simulink library "Nokia_Arduino_Blocks"  (Simulink 7.5)
settings: Solver=ode45  StartTime=0.0  StopTime=10.0  RelTol=1e-3
settings Model: Creator=tyler  LastModifiedBy=Wildcat

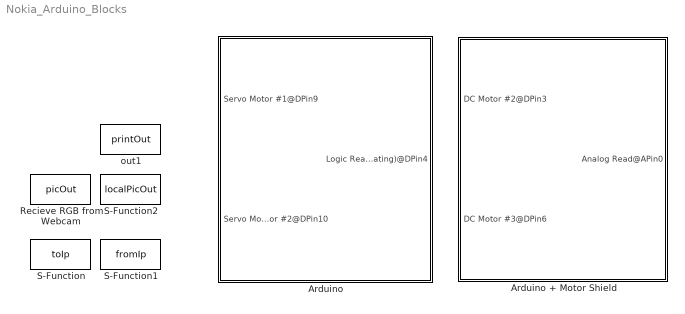
== system Nokia_Arduino_Blocks ==
  Arduino : Subsystem  mask{PinConfig0=Rx, PinConfig1=Tx, PinConfig2=Unused, PinConfig3=Unused, PinConfig4=Logic Read (floating), PinConfig5=Unused, PinConfig6=Unused, PinConfig7=Unused, PinConfig8=Unused, PinConfig9=Servo Motor #1, PinConfig10=Servo Motor #2, PinConfig11=Unused, PinConfig12=Unused, PinConfig13=Unused, ApinConfig0=Unused, ApinConfig1=Unused, ApinConfig2=Unused, ApinConfig3=Unused, ApinConfig4=Unused, ApinConfig5=Unused}
      mask prompts: PinConfig0 "Digital Pin 0 :"; PinConfig1 "Digital Pin 1 :"; PinConfig2 "Digital Pin 2 :"; PinConfig3 "Digital Pin 3 :"; PinConfig4 "Digital Pin 4 :"; PinConfig5 "Digital Pin 5 :"; PinConfig6 "Digital Pin 6 :"; PinConfig7 "Digital Pin 7 :"; PinConfig8 "Digital Pin 8 :"; PinConfig9 "Digital Pin 9 :"; PinConfig10 "Digital Pin 10:"; PinConfig11 "Digital Pin 11:"; PinConfig12 "Digital Pin 12:"; PinConfig13 "Digital Pin 13:"; ApinConfig0 "Analog Input 0:"; ApinConfig1 "Analog Input 1:"; ApinConfig2 "Analog Input 2:"; ApinConfig3 "Analog Input 3:"; ApinConfig4 "Analog Input 4:"; ApinConfig5 "Analog Input 5:"
      mask init:
      | set_param(gcb, 'LinkStatus', 'none')
      | ardInterface('all');
      mask StyleString: popup(Unused|Rx|Logic Write|Logic Read (floating)|Logic Read (pulled high)),popup(Unused|Tx|Logic Write|Logic Read (floating)|Logic Read (pulled high)),popup(Unused|Encoder (with pin 4)|Logic Write|Logic Read (floating)|Logic Read (pulled high)),popup(Unused|Encoder (with pin 5)|PWM Write|Logic Write|Logic Read (floating)|Logic Read (pulled high)),popup(Unused|Logic Write|Logic Read (floating)|Logic Read (pulled high)),popup(Unused|PWM Write|Logic Write|Logic Read (floating)|Logic Read (pulled high)),popup(Unused|PWM Write|Logic Write|Logic Read (floating)|Logic Read (pulled high)),popup(Unused|Logic Write|Logic Read (floating)|Logic Read (pulled high)),popup(Unused|Logic Write|Logic Read (floating)|Logic Read (pulled high)),popup(Unused|PWM Write|Logic Write|Servo Motor #1|Logic Read (floating)|Logic Read (pulled high)),popup(Unused|PWM Write|Logic Write|Servo Motor #2|Logic Read (floating)|Logic Read (pulled high)),popup(Unused|PWM Write|Logic Write|Logic Read (floating)|Logic Read (pulled high)),popup(Unused|PWM Write|Logic Write|Logic Read (floating)|Logic Read (pulled high)),popup(Unused|Logic Write|Logic Read (floating)|Logic Read (pulled high)),popup(Unused|Analog Read),popup(Unused|Analog Read),popup(Unused|Analog Read),popup(Unused|Analog Read),popup(Unused|Analog Read),popup(Unused|Analog Read)
      mask CallbackString:
      | ||ardInterface('clearAll');
      | set_param(gcb, 'LinkStatus', 'none')
      | maskStr = get_param(gcb,'MaskEnables');
      | maskVals = get_param(gcb,'MaskValues');
      | if strcmp(get_param(gcb,'PinConfig2'),'Encoder (with pin 4)')
      |     maskStr{5}='off';
      |     maskVals{5}='Unused';
      | else
      |     maskStr{5}='on';
      | end
      | 
      | set_param(gcb,'MaskEnables',maskStr);
      | set_param(gcb,'MaskValues',maskVals);
      | |ardInterface('clearAll');
      | set_param(gcb, 'LinkStatus', 'none')
      | maskStr = get_param(gcb,'MaskEnables');
      | maskVals = get_param(gcb,'MaskValues');
      | if strcmp(get_param(gcb,'PinConfig3'),'Encoder (with pin 5)')
      |     maskStr{6}='off';
      |     maskVals{6}='Unused';
      | else
      |     maskStr{6}='on';
      | end
      | 
      | set_param(gcb,'MaskEnables',maskStr);
      | set_param(gcb,'MaskValues',maskVals);
      | ||||||||||||||||
      mask TabNameString: Digital I/O,Digital I/O,Digital I/O,Digital I/O,Digital I/O,Digital I/O,Digital I/O,Digital I/O,Digital I/O,Digital I/O,Digital I/O,Digital I/O,Digital I/O,Digital I/O,Analog Output,Analog Output,Analog Output,Analog Output,Analog Output,Analog Output
  Arduino + Motor Shield : Subsystem  mask{PinConfig0=Rx, PinConfig1=Tx, PinConfig2=Unused, PinConfig3=DC Motor #2, PinConfig4=Unused, PinConfig5=Unused, PinConfig6=DC Motor #3, PinConfig7=Unused, PinConfig8=Unused, PinConfig9=Unused, PinConfig10=Unused, PinConfig11=Unused, PinConfig12=Unused, PinConfig13=Unused, ApinConfig0=Analog Read, ApinConfig1=Unused, ApinConfig2=Unused, ApinConfig3=Unused, ApinConfig4=Unused, ApinConfig5=Unused}
      mask prompts: PinConfig0 "Digital Pin 0 :"; PinConfig1 "Digital Pin 1 :"; PinConfig2 "Digital Pin 2 :"; PinConfig3 "Digital Pin 3 :"; PinConfig4 "Digital Pin 4 :"; PinConfig5 "Digital Pin 5 :"; PinConfig6 "Digital Pin 6 :"; PinConfig7 "Digital Pin 7 :"; PinConfig8 "Digital Pin 8 :"; PinConfig9 "Digital Pin 9 :"; PinConfig10 "Digital Pin 10:"; PinConfig11 "Digital Pin 11:"; PinConfig12 "Digital Pin 12:"; PinConfig13 "Digital Pin 13:"; ApinConfig0 "Analog Input 0:"; ApinConfig1 "Analog Input 1:"; ApinConfig2 "Analog Input 2:"; ApinConfig3 "Analog Input 3:"; ApinConfig4 "Analog Input 4:"; ApinConfig5 "Analog Input 5:"
      mask init:
      | set_param(gcb, 'LinkStatus', 'none')
      | ardInterface('all');
      mask StyleString: popup(Unused|Rx|Logic Write|Logic Read (floating)|Logic Read (pulled high)),popup(Unused|Tx|Logic Write|Logic Read (floating)|Logic Read (pulled high)),popup(Unused|Encoder (with pin 9)|Logic Write|Logic Read (floating)|Logic Read (pulled high)),popup(Unused|Encoder (with pin 10)|PWM Write|Logic Write|Logic Read (floating)|Logic Read (pulled high)|DC Motor #2|Stepper Motor #1),popup(Unused|Logic Write|Logic Read (floating)|Logic Read (pulled high)),popup(Unused|PWM Write|Logic Write|Logic Read (floating)|Logic Read (pulled high)|DC Motor #4|Stepper Motor #2),popup(Unused|PWM Write|Logic Write|Logic Read (floating)|Logic Read (pulled high)|DC Motor #3|Stepper Motor #2),popup(Unused|Logic Write|Logic Read (floating)|Logic Read (pulled high)),popup(Unused|Logic Write|Logic Read (floating)|Logic Read (pulled high)),popup(Unused|PWM Write|Logic Write|Logic Read (floating)|Logic Read (pulled high)),popup(Unused|PWM Write|Logic Write|Logic Read (floating)|Logic Read (pulled high)),popup(Unused|PWM Write|Logic Write|Logic Read (floating)|Logic Read (pulled high)|DC Motor #1|Stepper Motor #1),popup(Unused|PWM Write|Logic Write|Logic Read (floating)|Logic Read (pulled high)),popup(Unused|Logic Write|Logic Read (floating)|Logic Read (pulled high)),popup(Unused|Analog Read),popup(Unused|Analog Read),popup(Unused|Analog Read),popup(Unused|Analog Read),popup(Unused|Analog Read),popup(Unused|Analog Read)
      mask CallbackString:
      | ardInterface('clearAll');|ardInterface('clearAll');|ardInterface('clearAll');
      | set_param(gcb, 'LinkStatus', 'none')
      | maskStr = get_param(gcb,'MaskEnables');
      | maskVals = get_param(gcb,'MaskValues');
      | if strcmp(get_param(gcb,'PinConfig2'),'Encoder (with pin 9)')
      |     maskStr{10}='off';
      |     maskVals{10}='Unused';
      | else
      |     maskStr{10}='on';
      | end
      | 
      | set_param(gcb,'MaskEnables',maskStr);
      | set_param(gcb,'MaskValues',maskVals);
      | |ardInterface('clearAll');
      | set_param(gcb, 'LinkStatus', 'none')
      | maskStr = get_param(gcb,'MaskEnables');
      | maskVals = get_param(gcb,'MaskValues');
      | if strcmp(get_param(gcb,'PinConfig3'),'Encoder (with pin 10)')
      |     maskStr{11}='off';
      |     maskVals{11}='Unused';
      | else
      |     maskStr{11}='on';
      | end
      | 
      | if strcmp(get_param(gcb,'PinConfig3'),'Stepper Motor #1')
      |     maskStr{12}='off';
      |     maskVals{12}='Unused';
      | else
      |     maskStr{12}='on';
      | end
      | if (sum(cell2mat(strfind(get_param(gcb,'MaskValues'),'Motor'))))
      | maskStr{5}='off';
      | maskVals{5}='Unused';
      | maskStr{8}='off';
      | maskVals{8}='Unused';
      | maskStr{9}='off';
      | maskVals{9}='Unused';
      | maskStr{13}='off';
      | maskVals{13}='Unused';
      | else
      | maskStr{5}='on';
      | maskStr{8}='on';
      | maskStr{9}='on';
      | maskStr{13}='on';
      | end
      | set_param(gcb,'MaskEnables',maskStr);
      | set_param(gcb,'MaskValues',maskVals);|ardInterface('clearAll');
      | |ardInterface('clearAll');
      | set_param(gcb, 'LinkStatus', 'none')
      | maskStr = get_param(gcb,'MaskEnables');
      | maskVals = get_param(gcb,'MaskValues');
      | if strcmp(get_param(gcb,'PinConfig5'),'Stepper Motor #2')
      |     maskStr{7}='off';
      |     maskVals{7}='Unused';
      | else
      |     maskStr{7}='on';
      | end
      | if (sum(cell2mat(strfind(get_param(gcb,'MaskValues'),'Motor'))))
      | maskStr{5}='off';
      | maskVals{5}='Unused';
      | maskStr{8}='off';
      | maskVals{8}='Unused';
      | maskStr{9}='off';
      | maskVals{9}='Unused';
      | maskStr{13}='off';
      | maskVals{13}='Unused';
      | else
      | maskStr{5}='on';
      | maskStr{8}='on';
      | maskStr{9}='on';
      | maskStr{13}='on';
      | end
      | set_param(gcb,'MaskEnables',maskStr);
      | set_param(gcb,'MaskValues',maskVals);|ardInterface('clearAll');
      | set_param(gcb, 'LinkStatus', 'none')
      | maskStr = get_param(gcb,'MaskEnables');
      | maskVals = get_param(gcb,'MaskValues');
      | maskVals = get_param(gcb,'MaskValues');
      | if strcmp(get_param(gcb,'PinConfig6'),'Stepper Motor #2')
      |     maskStr{6}='off';
      |     maskVals{6}='Unused';
      | else
      |     maskStr{6}='on';
      | end
      | if (sum(cell2mat(strfind(get_param(gcb,'MaskValues'),'Motor'))))
      | maskStr{5}='off';
      | maskVals{5}='Unused';
      | maskStr{8}='off';
      | maskVals{8}='Unused';
      | maskStr{9}='off';
      | maskVals{9}='Unused';
      | maskStr{13}='off';
      | maskVals{13}='Unused';
      | else
      | maskStr{5}='on';
      | maskStr{8}='on';
      | maskStr{9}='on';
      | maskStr{13}='on';
      | end
      | set_param(gcb,'MaskEnables',maskStr);
      | set_param(gcb,'MaskValues',maskVals);|ardInterface('clearAll');
      | |ardInterface('clearAll');
      | set_param(gcb, 'LinkStatus', 'none')
      | maskStr = get_param(gcb,'MaskEnables');
      | maskVals = get_param(gcb,'MaskValues');
      | if (sum(cell2mat(strfind(get_param(gcb,'MaskValues'),'Motor'))))
      | maskStr{5}='off';
      | maskVals{5}='Unused';
      | maskStr{8}='off';
      | maskVals{8}='Unused';
      | maskStr{9}='off';
      | maskVals{9}='Unused';
      | maskStr{13}='off';
      | maskVals{13}='Unused';
      | else
      | maskStr{5}='on';
      | maskStr{8}='on';
      | maskStr{9}='on';
      | maskStr{13}='on';
      | end
      | set_param(gcb,'MaskEnables',maskStr);
      | set_param(gcb,'MaskValues',maskVals);|ardInterface('clearAll');
      | |ardInterface('clearAll');
      | set_param(gcb, 'LinkStatus', 'none')
      | maskStr = get_param(gcb,'MaskEnables');
      | maskVals = get_param(gcb,'MaskValues');
      | if (sum(cell2mat(strfind(get_param(gcb,'MaskValues'),'Motor'))))
      | maskStr{5}='off';
      | maskVals{5}='Unused';
      | maskStr{8}='off';
      | maskVals{8}='Unused';
      | maskStr{9}='off';
      | maskVals{9}='Unused';
      | maskStr{13}='off';
      | maskVals{13}='Unused';
      | else
      | maskStr{5}='on';
      | maskStr{8}='on';
      | maskStr{9}='on';
      | maskStr{13}='on';
      | end
      | set_param(gcb,'MaskEnables',maskStr);
      | set_param(gcb,'MaskValues',maskVals);|ardInterface('clearAll');
      | set_param(gcb, 'LinkStatus', 'none')
      | maskStr = get_param(gcb,'MaskEnables');
      | maskVals = get_param(gcb,'MaskValues');
      | if strcmp(get_param(gcb,'PinConfig11'),'Stepper Motor #1')
      |     maskStr{4}='off';
      |     maskVals{4}='Unused';
      | else
      |     maskStr{4}='on';
      | end
      | if (sum(cell2mat(strfind(get_param(gcb,'MaskValues'),'Motor'))))
      | maskStr{5}='off';
      | maskVals{5}='Unused';
      | maskStr{8}='off';
      | maskVals{8}='Unused';
      | maskStr{9}='off';
      | maskVals{9}='Unused';
      | maskStr{13}='off';
      | maskVals{13}='Unused';
      | else
      | maskStr{5}='on';
      | maskStr{8}='on';
      | maskStr{9}='on';
      | maskStr{13}='on';
      | end
      | set_param(gcb,'MaskEnables',maskStr);
      | set_param(gcb,'MaskValues',maskVals);|ardInterface('clearAll');
      | |ardInterface('clearAll');
      | |ardInterface('clearAll');
      | |ardInterface('clearAll');
      | |ardInterface('clearAll');
      | |ardInterface('clearAll');
      | |ardInterface('clearAll');
      | |ardInterface('clearAll');
      mask TabNameString: Digital I/O,Digital I/O,Digital I/O,Digital I/O,Digital I/O,Digital I/O,Digital I/O,Digital I/O,Digital I/O,Digital I/O,Digital I/O,Digital I/O,Digital I/O,Digital I/O,Analog Output,Analog Output,Analog Output,Analog Output,Analog Output,Analog Output
  Recieve RGB from Webcam : S-Function  FunctionName=picOut  Parameters=153 104 42 82  EnableBusSupport=off
  S-Function : S-Function  FunctionName=toIp  Parameters='153.104.47.61','6667'  EnableBusSupport=off
  S-Function1 : S-Function  FunctionName=fromIp  Parameters='6667' 0  EnableBusSupport=off
  S-Function2 : S-Function  FunctionName=localPicOut  Parameters=320 240 320 240  EnableBusSupport=off
  out1 : S-Function  FunctionName=printOut  EnableBusSupport=off

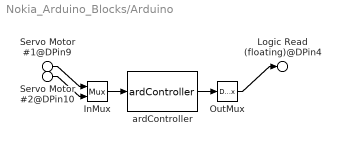
== system Nokia_Arduino_Blocks/Arduino ==
  Servo Motor #1@DPin9 : Inport
  Servo Motor #2@DPin10 : Inport  Port=2
  InMux : Mux  Inputs=2
  OutMux : Demux  Outputs=1
  ardController : S-Function  FunctionName=ardController  Parameters='[:D4F:M1S:M2S]' '2' '1'  EnableBusSupport=off
  Logic Read (floating)@DPin4 : Outport
  wires:
  InMux/1 -> ardController/1
  ardController/1 -> OutMux/1
  OutMux/1 -> Logic Read (floating)@DPin4/1
  Servo Motor #1@DPin9/1 -> InMux/1
  Servo Motor #2@DPin10/1 -> InMux/2

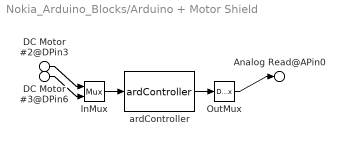
== system Nokia_Arduino_Blocks/Arduino + Motor Shield ==
  DC Motor #2@DPin3 : Inport
  DC Motor #3@DPin6 : Inport  Port=2
  InMux : Mux  Inputs=2
  OutMux : Demux  Outputs=1
  ardController : S-Function  FunctionName=ardController  Parameters='[:M2M:M3M:A0A]' '2' '1'  EnableBusSupport=off
  Analog Read@APin0 : Outport
  wires:
  InMux/1 -> ardController/1
  ardController/1 -> OutMux/1
  DC Motor #2@DPin3/1 -> InMux/1
  DC Motor #3@DPin6/1 -> InMux/2
  OutMux/1 -> Analog Read@APin0/1
